simulink model "CessnaSimClosed"  (R2017b)
settings: Solver=VariableStepAuto  StartTime=0.0  StopTime=10.0  RelTol=1e-3
values from neighbouring files (symbols this model uses):
  alpha0 = 0    [Cessna_Simulation.m]
  CDM = 0.0223    [Cessna_Simulation.m]
  CL0 = 0.307    [Cessna_Simulation.m]
  CLa = 4.41    [Cessna_Simulation.m]
  CLadot = 1.7    [Cessna_Simulation.m]
  CLDM = 0    [Cessna_Simulation.m]
  CLel = 0.43    [Cessna_Simulation.m]
  CLq = 3.9    [Cessna_Simulation.m]
  CMadot = -7.27    [Cessna_Simulation.m]
  CMel = -1.122    [Cessna_Simulation.m]
  CMq = -12.4    [Cessna_Simulation.m]
  eta = 0    [Cessna_Simulation.m]
  k = 0.0554    [Cessna_Simulation.m]
  m = W/g    (= 82.298136646)    [Cessna_Simulation.m]
  q0 = 0    [Cessna_Simulation.m]
  rho = 2.377*10^-3    (= 0.002377)    [Cessna_Simulation.m]
  S = 174    [Cessna_Simulation.m]
  theta0 = 0    [Cessna_Simulation.m]
  V0 = 140    [Cessna_Simulation.m]
  W = 2650    [Cessna_Simulation.m]
  x0 = [V0;alpha0;theta0;q0;0]    [Cessna_Simulation.m]
undefined symbols (not defined in the file or in its folder): cbar, CM0, CMa, J2, magnitude
settings Model: Creator=stroll  LastModifiedBy=stroll

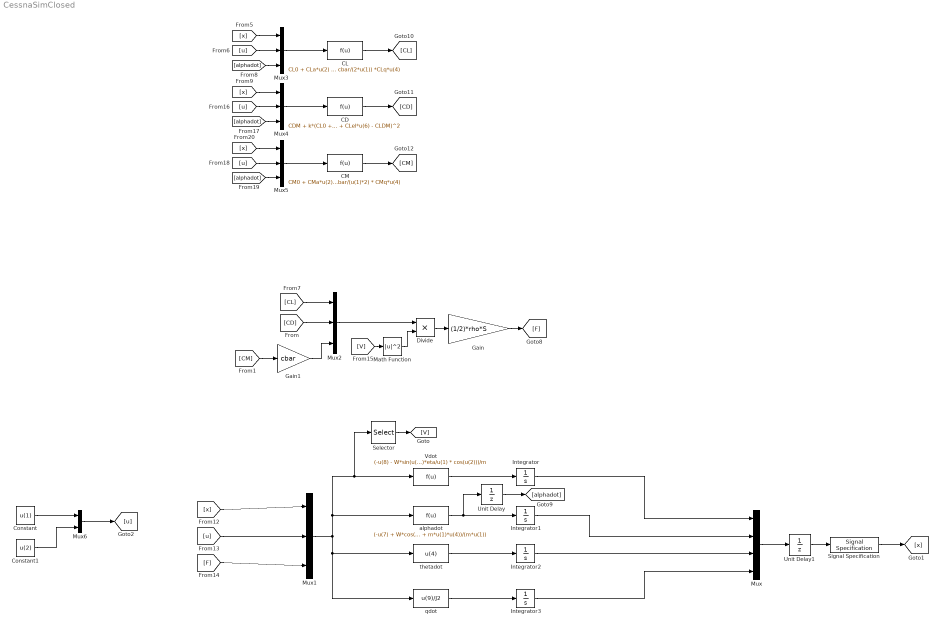
== system CessnaSimClosed ==
  CD : Fcn  Expr=CDM + k*(CL0 + CLa*u(2) + CLel*u(6) - CLDM)^2
  CL : Fcn  Expr=CL0 + CLa*u(2) + CLel*u(6) + cbar/(2*u(1))*CLadot*u(7) + cbar/(2*u(1)) *CLq*u(4)
  CM : Fcn  Expr=CM0 + CMa*u(2) + CMel*u(6) + cbar/(u(1)*2) * CMadot*u(7) + cbar/(u(1)*2) * CMq*u(4)
  Constant : Constant  Value=u(1)
  Constant1 : Constant  Value=u(2)
  Divide : Product  Inputs=**
  Gain : Gain  Gain=(1/2)*rho*S
  Gain1 : Gain  Gain=cbar
  Integrator : Integrator  InitialCondition=V0
  Integrator1 : Integrator  InitialCondition=alpha0
  Integrator2 : Integrator  InitialCondition=theta0
  Integrator3 : Integrator  InitialCondition=q0
  Math Function : Math  Operator=magnitude^2  SaturateOnIntegerOverflow=on
  Mux : Mux
  Mux{1..5} (5 alike) : Mux  Inputs=3
  Mux6 : Mux  Inputs=2
  Selector : Selector  InputPortWidth=3  IndexOptions=Index vector (dialog)  Indices=[1]  OutputSizes=1
  Signal Specification : SignalSpecification  Dimensions=[4,1]
  Unit Delay : UnitDelay  SampleTime=-1
  Unit Delay1 : UnitDelay  InitialCondition=x0  SampleTime=-1
  Vdot : Fcn  Expr=(-u(8) - W*sin(u(3)-u(2)) + 550*u(5)*eta/u(1) * cos(u(2)))/m
  alphadot : Fcn  Expr=(-u(7) + W*cos(u(3)-u(2)) - (550*u(5)*eta/u(1))*sin(u(2)) + m*u(1)*u(4))/(m*u(1))
  qdot : Fcn  Expr=u(9)/J2
  thetadot : Fcn  Expr=u(4)
  wires:
  CM/1 -> [CM]
  [u] -> Mux5/2
  Mux3/1 -> CL/1
  [CM] -> Gain1/1
  [u] -> Mux3/2
  Integrator1/1 -> Mux/2
  [x] -> Mux1/1
  alphadot/1 -> Unit Delay/1, Integrator1/1
  Vdot/1 -> Integrator/1
  [alphadot] -> Mux3/3
  Integrator/1 -> Mux/1
  [alphadot] -> Mux5/3
  [V] -> Math Function/1
  Integrator2/1 -> Mux/3
  Mux5/1 -> CM/1
  thetadot/1 -> Integrator2/1
  Gain1/1 -> Mux2/3
  Integrator3/1 -> Mux/4
  [CD] -> Mux2/2
  qdot/1 -> Integrator3/1
  [F] -> Mux1/3
  [CL] -> Mux2/1
  Unit Delay/1 -> [alphadot]
  [x] -> Mux5/1
  Mux2/1 -> Divide/1
  CD/1 -> [CD]
  Divide/1 -> Gain/1
  [x] -> Mux4/1
  [u] -> Mux4/2
  [alphadot] -> Mux4/3
  [x] -> Mux3/1
  [u] -> Mux1/2
  CL/1 -> [CL]
  Mux4/1 -> CD/1
  Math Function/1 -> Divide/2
  Gain/1 -> [F]
  Mux1/1 -> qdot/1, thetadot/1, alphadot/1, Selector/1, Vdot/1
  Mux/1 -> Unit Delay1/1
  Unit Delay1/1 -> Signal Specification/1
  Signal Specification/1 -> [x]
  Selector/1 -> [V]
  Constant/1 -> Mux6/1
  Constant1/1 -> Mux6/2
  Mux6/1 -> [u]
